simulink model "AvailableCoins"  (R2023a)
settings: Solver=FixedStepAuto  StartTime=0.0  StopTime=Inf  RelTol=1e-3  SampleTimeConstraint=STIndependent
undefined symbols (not defined in the file): AVAILABLE_COINS_REGISTER, BIT_MASK_010_CENTS, BIT_MASK_020_CENTS, BIT_MASK_050_CENTS, BIT_MASK_100_CENTS, BIT_MASK_ADD_LED, BIT_MASK_BOTH_LEDS_NOT, BIT_MASK_RETURN_LED, char2dec, PERIPHERALS_REGISTER
libraries: simulink x8
Description:
  | % Copyright 2023 The MathWorks, Inc.
settings Model: DataDictionary=Parameters.sldd  EnableAccessToBaseWorkspace=off  Creator=sdupertu  LastModifiedBy=sdupertu
settings SolverCC: AlgebraicLoopSolver=TrustRegion
settings DataIOCC: SaveOutput=off  SaveTime=off
settings OptimizationCC: DefaultParameterBehavior=Inlined  EnhancedBackFolding=on  PassReuseOutputArgsAs=Individual arguments  OptimizeBlockOrder=speed  DifferentSizesBufferReuse=on  OptimizationCustomize=off  EfficientTunableParamExpr=on
settings DebuggingCC: ParameterTunabilityLossMsg=error  UnconnectedInputMsg=warning  UnconnectedOutputMsg=warning  UnconnectedLineMsg=warning  PregeneratedLibrarySubsystemCodeDiagnostic=none  ArithmeticOperatorsInVariantConditions=warning
settings ModelReferenceCC: EnableRefExpFcnMdlSchedulingChecks=on  EnableParallelModelReferenceBuilds=on
settings SFSimCC: SimUseLocalCustomCode=off  MATLABDynamicMemAlloc=off  CustomCodeUndefinedFunction=UseInterfaceOnly
settings RTWCC: Description=Embedded Coder  SystemTargetFile=ert.tlc  TemplateMakefile=ert_default_tmf  RTWUseLocalCustomCode=off  IncludeHyperlinkInReport=on  DLArmComputeVersion=19.05
settings CodeAppCC: ForceParamTrailComments=on  IgnoreCustomStorageClasses=off  MaxIdLength=61  OperatorAnnotations=on  SimulinkDataObjDesc=on  SFDataObjDesc=on  InsertBlockDesc=on
settings ERTTargetCC: TargetLangStandard=C99 (ISO)  GenerateSampleERTMain=on  InlinedParameterPlacement=NonHierarchical  ERTCustomFileTemplate=example_file_process.tlc

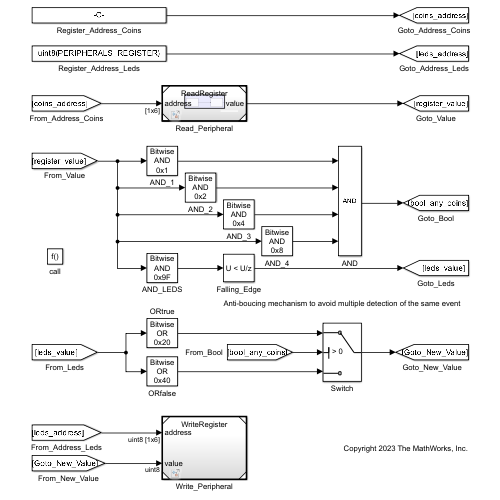
[thumbnail: Simulink's stored preview of the top-level diagram]
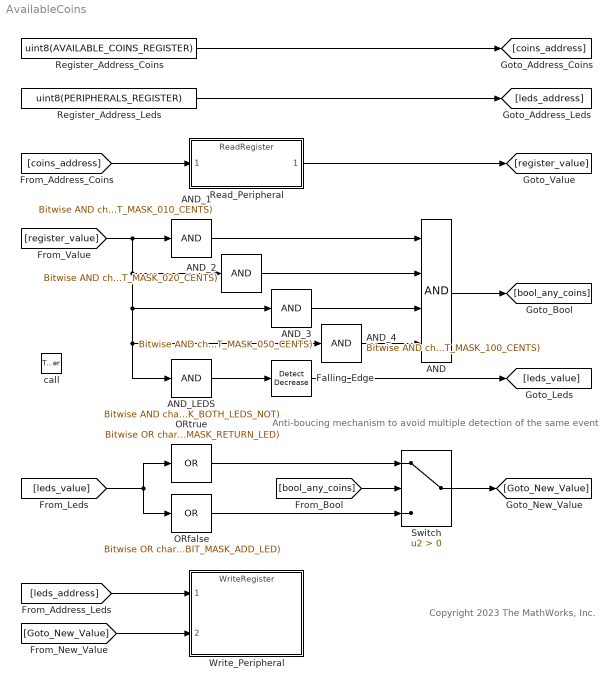
== system AvailableCoins ==
  note: Copyright 2023 The MathWorks, Inc.
  note: Anti-boucing mechanism to avoid multiple detection of the same event
  call : TriggerPort  TriggerType=function-call  VariantControl=Variant  PortDimensions=1  TriggerSignalSampleTime=[0.001,0]
  AND : Logic  Inputs=4  AllPortsSameDT=off  OutDataTypeStr=boolean
  AND_1 : simulink/Logic and Bit Operations/Bitwise Operator  logicop=AND  UseBitMask=on  BitMask=char2dec(BIT_MASK_010_CENTS)  BitMaskRealWorld=Stored Integer
  AND_2 : simulink/Logic and Bit Operations/Bitwise Operator  logicop=AND  UseBitMask=on  BitMask=char2dec(BIT_MASK_020_CENTS)  BitMaskRealWorld=Stored Integer
  AND_3 : simulink/Logic and Bit Operations/Bitwise Operator  logicop=AND  UseBitMask=on  BitMask=char2dec(BIT_MASK_050_CENTS)  BitMaskRealWorld=Stored Integer
  AND_4 : simulink/Logic and Bit Operations/Bitwise Operator  logicop=AND  UseBitMask=on  BitMask=char2dec(BIT_MASK_100_CENTS)  BitMaskRealWorld=Stored Integer
  AND_LEDS : simulink/Logic and Bit Operations/Bitwise Operator  logicop=AND  UseBitMask=on  BitMask=char2dec(BIT_MASK_BOTH_LEDS_NOT)  BitMaskRealWorld=Stored Integer
  Falling_Edge : simulink/Logic and Bit Operations/Detect Decrease  vinit=0  OutDataTypeStr=uint8
  ORfalse : simulink/Logic and Bit Operations/Bitwise Operator  logicop=OR  UseBitMask=on  BitMask=char2dec(BIT_MASK_ADD_LED)  BitMaskRealWorld=Stored Integer
  ORtrue : simulink/Logic and Bit Operations/Bitwise Operator  logicop=OR  UseBitMask=on  BitMask=char2dec(BIT_MASK_RETURN_LED)  BitMaskRealWorld=Stored Integer
  Read_Peripheral : ModelReference  ModelNameDialog=ReadRegister  SimulationMode=Normal  ModelReferenceVersion=8.12
  Register_Address_Coins : Constant  Value=uint8(AVAILABLE_COINS_REGISTER)  SampleTime=-1
  Register_Address_Leds : Constant  Value=uint8(PERIPHERALS_REGISTER)  SampleTime=-1
  Switch : Switch  Criteria=u2 > Threshold  SaturateOnIntegerOverflow=off  InputSameDT=off
  Write_Peripheral : ModelReference  ModelNameDialog=WriteRegister  SimulationMode=Normal  ModelReferenceVersion=8.7
  wires:
  Register_Address_Coins/1 -> [coins_address]
  [leds_address] -> Write_Peripheral/1
  [coins_address] -> Read_Peripheral/1
  Read_Peripheral/1 -> [register_value]
  [Goto_New_Value] -> Write_Peripheral/2
  AND_1/1 -> AND/1
  [register_value] -> AND_1/1, AND_2/1, AND_3/1, AND_4/1, AND_LEDS/1
  AND_3/1 -> AND/3
  AND_2/1 -> AND/2
  AND_4/1 -> AND/4
  AND/1 -> [bool_any_coins]
  AND_LEDS/1 -> Falling_Edge/1
  Register_Address_Leds/1 -> [leds_address]
  Falling_Edge/1 -> [leds_value]
  ORfalse/1 -> Switch/3
  [bool_any_coins] -> Switch/2
  [leds_value] -> ORtrue/1, ORfalse/1
  Switch/1 -> [Goto_New_Value]
  ORtrue/1 -> Switch/1
